simulink model "sampleModel1492_3_sub"  (R2023a)
settings: Solver=VariableStepAuto  StartTime=0.0  StopTime=10.0  RelTol=1e-3
libraries: hdlsllib x5, simulink x1
settings Model: Creator=user1  LastModifiedBy=user1
settings OptimizationCC: BlockReduction=off  ConditionallyExecuteInputs=off

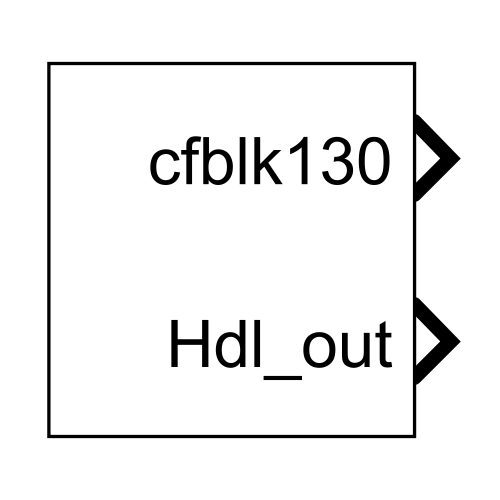
[thumbnail: Simulink's stored preview of the top-level diagram]
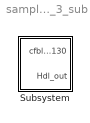
== system sampleModel1492_3_sub ==
  Subsystem : Subsystem

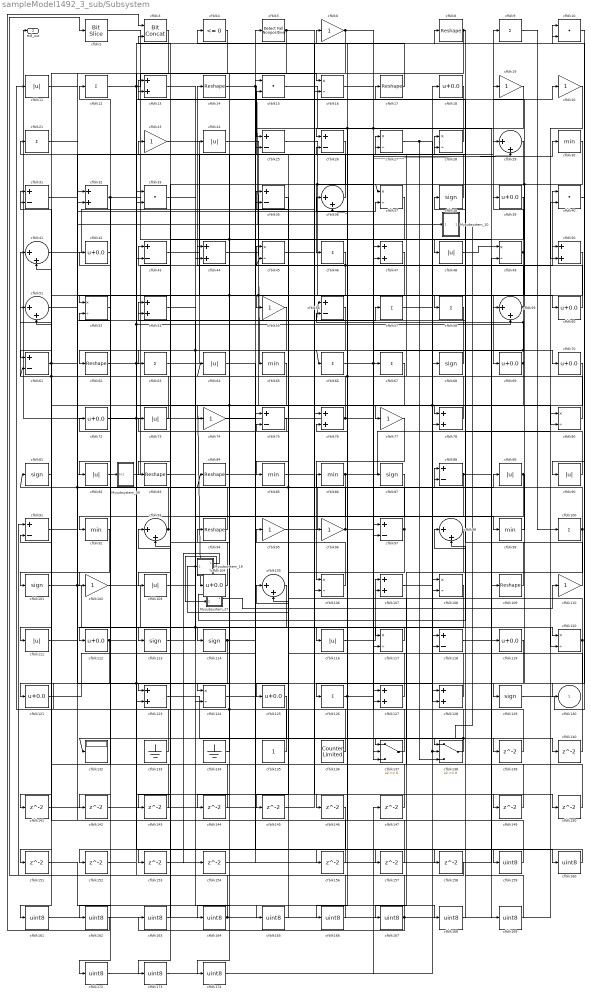
== system sampleModel1492_3_sub/Subsystem ==
  Mysubsystem_10 : Subsystem  TreatAsAtomicUnit=on  RTWFcnName=Mysubsystem_10
      settings: RTWFcnNameOpts=User specified  RTWFileNameOpts=Use function name
  Mysubsystem_19 : Subsystem  TreatAsAtomicUnit=on  RTWFcnName=Mysubsystem_19
      settings: RTWFcnNameOpts=User specified  RTWFileNameOpts=Use function name
  Mysubsystem_27 : Subsystem  TreatAsAtomicUnit=on  RTWFcnName=Mysubsystem_27
      settings: RTWFcnNameOpts=User specified  RTWFileNameOpts=Use function name
  Mysubsystem_39 : Subsystem  TreatAsAtomicUnit=on  RTWFcnName=Mysubsystem_39
      settings: RTWFcnNameOpts=User specified  RTWFileNameOpts=Use function name
  cfblk{10,15,33,40} (4 alike) : DotProduct  OutDataTypeStr=uint8
  cfblk{9,12,21,46,57..58,63,66..67,100,126} (11 alike) : Sum  Inputs=+  OutDataTypeStr=uint8
  cfblk{38,68,81,87,101,113..114,129} (8 alike) : Signum
  cfblk{6,19..20,23,55,74,77,95..96,102,110} (11 alike) : Gain  OutDataTypeStr=uint8
  cfblk{11,24,48,64,73,82,89..90,103,111,116} (11 alike) : Abs  OutDataTypeStr=uint8  SaturateOnIntegerOverflow=off
  cfblk{18,39,42,60,69..70,72,104,112,119,121,125} (12 alike) : Bias  Bias=0.0  SaturateOnIntegerOverflow=off
  cfblk{29,36,41,51,59,93,98,105} (8 alike) : Sum  Inputs=|++  OutDataTypeStr=uint8
  cfblk{16,27..28,37,45,49,52,80,106,108,117,120,124} (13 alike) : Product  Inputs=*/  OutDataTypeStr=uint8  RndMeth=Zero  SaturateOnIntegerOverflow=on
  cfblk{13,32,44,47,50,53,76,78,107,123,127..128} (12 alike) : Sum  OutDataTypeStr=uint8
  cfblk{8,14,17,62,83..84,94,109} (8 alike) : Reshape
  cfblk{25..26,31,35,43,56,61,75,88,91,97,118} (12 alike) : Sum  Inputs=+-  OutDataTypeStr=uint8
  cfblk132 : Display
  cfblk133 : Ground
  cfblk134 : Ground
  cfblk135 : Constant  OutDataTypeStr=uint8  SampleTime=-1
  cfblk136 : hdlsllib/Sources/Counter Limited  uplimit=7  tsamp=-1
  cfblk137 : Switch  OutDataTypeStr=uint8  SaturateOnIntegerOverflow=off  InputSameDT=off
  cfblk138 : Switch  OutDataTypeStr=uint8  SaturateOnIntegerOverflow=off  InputSameDT=off
  cfblk{139..147,149..154,156..158} (18 alike) : Delay  SampleTime=1
  cfblk{159..169,172..174} (14 alike) : DataTypeConversion  OutDataTypeStr=uint8  SaturateOnIntegerOverflow=off  RndMeth=Floor
  cfblk2 : hdlsllib/Logic and Bit Operations/Bit Slice  lidx=7  ridx=0
  cfblk3 : hdlsllib/Logic and Bit Operations/Bit Concat  numInputs=2
  cfblk{30,65,85..86,92,99} (6 alike) : MinMax  OutDataTypeStr=uint8
  cfblk4 : hdlsllib/Logic and Bit Operations/Compare To Zero  relop=<=  OutDataTypeStr=uint8
  cfblk5 : hdlsllib/Logic and Bit Operations/Detect Fall Nonpositive  vinit=0  OutDataTypeStr=uint8
  cfblk130 : Outport  OutDataTypeStr=uint8  VectorParamsAs1DForOutWhenUnconnected=off
  Hdl_out : Outport  Port=2  OutDataTypeStr=uint8
  wires:
  cfblk73/1 -> cfblk41/1
  cfblk9/1 -> cfblk100/1
  cfblk102/1 -> cfblk114/1
  cfblk44/1 -> cfblk97/2, cfblk77/1
  cfblk25/1 -> cfblk87/1, cfblk58/1
  cfblk75/1 -> cfblk43/1
  cfblk6/1 -> cfblk70/1, cfblk61/1
  cfblk61/1 -> cfblk28/1, cfblk121/1
  cfblk36/1 -> cfblk21/1
  cfblk76/1 -> Hdl_out/1, cfblk31/2, cfblk29/2, cfblk67/1
  cfblk50/1 -> cfblk52/1
  cfblk112/1 -> cfblk88/2, cfblk11/1
  cfblk93/1 -> cfblk23/1, cfblk12/1
  cfblk29/1 -> cfblk46/1
  cfblk30/1 -> cfblk59/1, cfblk37/1
  cfblk19/1 -> cfblk26/1
  cfblk46/1 -> cfblk45/2, cfblk144/1, cfblk111/1
  cfblk63/1 -> cfblk27/1
  cfblk133/1 -> cfblk51/1
  cfblk42/1 -> cfblk82/1
  cfblk120/1 -> cfblk45/1, cfblk126/1
  cfblk72/1 -> cfblk156/1, cfblk59/2, cfblk20/1
  cfblk32/1 -> cfblk44/2, cfblk112/1
  cfblk114/1 -> cfblk160/1, cfblk151/1, cfblk123/2
  cfblk18/1 -> cfblk137/3, cfblk166/1, cfblk35/2
  cfblk59/1 -> cfblk25/2, cfblk78/1, cfblk56/1
  cfblk95/1 -> cfblk89/1
  cfblk48/1 -> cfblk49/1
  cfblk77/1 -> cfblk106/1
  cfblk13/1 -> cfblk158/1, cfblk117/2
  cfblk15/1 -> cfblk119/1
  cfblk105/1 -> cfblk164/1
  cfblk94/1 -> cfblk31/1, cfblk61/2
  cfblk82/1 -> cfblk40/1
  cfblk27/1 -> cfblk138/3, cfblk68/1
  cfblk92/1 -> cfblk101/1
  cfblk4/1 -> cfblk32/2
  cfblk121/1 -> cfblk5/1
  cfblk89/1 -> cfblk137/2, cfblk129/1
  cfblk111/1 -> cfblk84/1, cfblk37/2
  cfblk87/1 -> cfblk96/1
  cfblk127/1 -> cfblk75/2
  cfblk2/1 -> cfblk109/1
  cfblk69/1 -> cfblk28/2, cfblk66/1, cfblk78/2, cfblk104/1
  cfblk123/1 -> cfblk138/1
  cfblk12/1 -> cfblk80/2, cfblk16/1
  cfblk116/1 -> cfblk107/1
  cfblk104/1 -> cfblk73/1
  cfblk90/1 -> cfblk38/1
  cfblk8/1 -> cfblk174/1, Mysubsystem_27/1(In1)
  cfblk101/1 -> cfblk120/2, cfblk116/1
  cfblk49/1 -> cfblk118/2, cfblk9/1
  cfblk88/1 -> cfblk103/1, cfblk50/1
  cfblk24/1 -> cfblk97/1
  cfblk81/1 -> cfblk51/2
  cfblk14/1 -> cfblk60/1, cfblk65/1
  cfblk74/1 -> cfblk15/1
  cfblk56/1 -> cfblk124/2, cfblk83/1
  cfblk43/1 -> cfblk69/1
  cfblk128/1 -> cfblk36/1
  cfblk135/1 -> cfblk94/1
  cfblk23/1 -> cfblk128/1
  cfblk113/1 -> cfblk88/1
  cfblk62/1 -> cfblk149/1, cfblk10/2, cfblk14/1
  cfblk66/1 -> cfblk30/1
  cfblk38/1 -> cfblk15/2
  cfblk3/1 -> cfblk161/1
  cfblk110/1 -> cfblk53/1
  cfblk119/1 -> cfblk137/1
  cfblk5/1 -> cfblk150/1, cfblk33/2
  cfblk52/1 -> cfblk92/1
  cfblk41/1 -> cfblk17/1
  cfblk91/1 -> cfblk57/1
  cfblk65/1 -> cfblk141/1, cfblk124/1
  cfblk31/1 -> cfblk55/1
  cfblk60/1 -> cfblk39/1
  cfblk26/1 -> cfblk93/2
  cfblk107/1 -> cfblk118/1
  cfblk129/1 -> cfblk10/1
  cfblk137/1 -> cfblk76/2
  cfblk126/1 -> cfblk6/1, cfblk47/2
  cfblk80/1 -> cfblk27/2
  cfblk100/1 -> cfblk117/1, cfblk35/1, cfblk81/1
  cfblk109/1 -> cfblk13/1
  cfblk103/1 -> cfblk56/2
  cfblk138/1 -> cfblk132/1, cfblk42/1
  cfblk57/1 -> cfblk120/1
  cfblk117/1 -> cfblk113/1
  cfblk10/1 -> cfblk90/1
  cfblk17/1 -> cfblk4/1
  cfblk39/1 -> cfblk123/1, cfblk74/1
  cfblk134/1 -> cfblk44/1
  cfblk68/1 -> cfblk62/1
  cfblk45/1 -> cfblk8/1
  cfblk51/1 -> cfblk127/2
  cfblk99/1 -> cfblk19/1
  cfblk98/1 -> cfblk167/1
  cfblk97/1 -> cfblk125/1, cfblk72/1
  cfblk53/1 -> cfblk99/1
  cfblk78/1 -> cfblk64/1, cfblk36/2
  cfblk106/1 -> cfblk95/1
  cfblk96/1 -> cfblk29/1, cfblk86/1
  cfblk136/1 -> cfblk24/1, cfblk13/2
  cfblk33/1 -> cfblk128/2
  cfblk40/1 -> cfblk130/1
  cfblk28/1 -> cfblk25/1
  cfblk16/1 -> cfblk48/1
  cfblk20/1 -> cfblk50/2
  cfblk47/1 -> cfblk63/1
  cfblk85/1 -> cfblk106/2
  cfblk58/1 -> cfblk85/1
  cfblk86/1 -> cfblk40/2, cfblk102/1
  cfblk139/1 -> cfblk127/1
  cfblk124/1 -> cfblk140/1
  cfblk140/1 -> cfblk47/1
  cfblk141/1 -> cfblk16/2
  cfblk67/1 -> cfblk142/1
  cfblk142/1 -> cfblk43/2
  cfblk55/1 -> cfblk143/1
  cfblk143/1 -> cfblk91/2
  cfblk144/1 -> cfblk52/2
  cfblk37/1 -> cfblk145/1
  cfblk145/1 -> cfblk76/1
  cfblk84/1 -> cfblk146/1
  cfblk147/1 -> cfblk53/2
  cfblk149/1 -> cfblk107/2
  cfblk150/1 -> cfblk93/1
  cfblk70/1 -> cfblk153/1
  cfblk153/1 -> cfblk49/2
  cfblk154/1 -> cfblk75/1
  cfblk156/1 -> cfblk32/1
  cfblk64/1 -> cfblk157/1
  cfblk157/1 -> cfblk41/2
  cfblk158/1 -> cfblk2/1
  cfblk152/1 -> cfblk159/1
  cfblk159/1 -> cfblk26/2
  cfblk160/1 -> cfblk152/1
  cfblk161/1 -> cfblk18/1, cfblk138/2
  cfblk146/1 -> cfblk162/1
  cfblk162/1 -> cfblk3/1
  cfblk163/1 -> cfblk3/2
  cfblk164/1 -> cfblk91/1, cfblk80/1
  cfblk83/1 -> cfblk165/1
  cfblk165/1 -> cfblk105/1
  cfblk166/1 -> cfblk105/2
  cfblk167/1 -> cfblk33/1, cfblk163/1
  cfblk151/1 -> cfblk168/1
  cfblk168/1 -> cfblk98/1
  cfblk118/1 -> cfblk169/1
  cfblk169/1 -> cfblk98/2
  cfblk108/1 -> cfblk172/1
  cfblk172/1 -> cfblk147/1
  cfblk125/1 -> cfblk173/1
  cfblk173/1 -> cfblk108/1
  cfblk174/1 -> cfblk108/2
  cfblk11/1 -> Mysubsystem_10/1(In1)
  Mysubsystem_10/1(Out1) -> cfblk139/1
  cfblk35/1 -> Mysubsystem_19/1(In1)
  Mysubsystem_19/1(Out1) -> cfblk154/1
  Mysubsystem_19/2(Out2) -> Mysubsystem_27/2(In2)
  Mysubsystem_27/1(Out1) -> cfblk110/1
  cfblk21/1 -> Mysubsystem_39/1(In1)

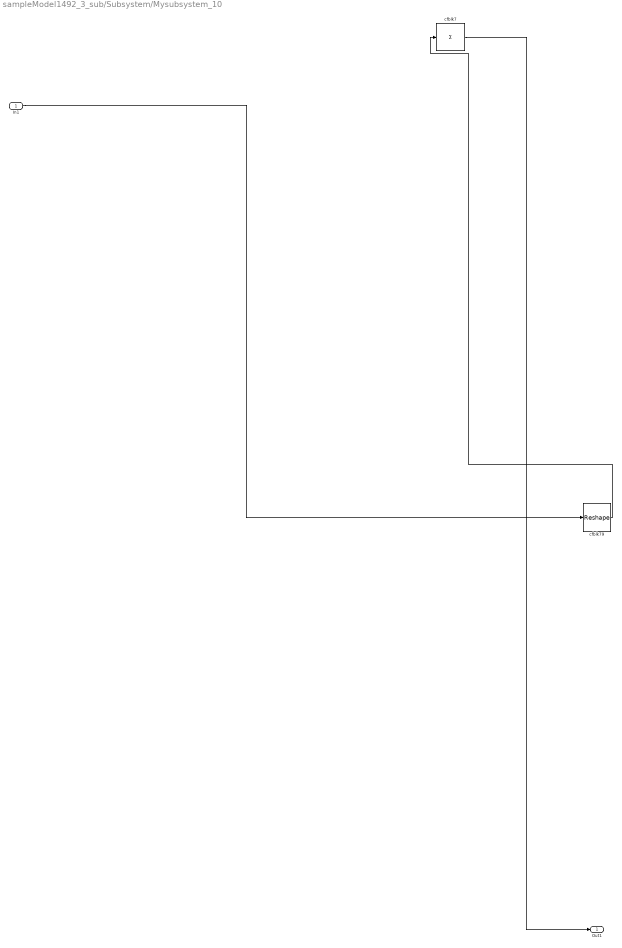
== system sampleModel1492_3_sub/Subsystem/Mysubsystem_10 ==
  In1 : Inport
  cfblk7 : Sum  Inputs=+
  cfblk79 : Reshape
  Out1 : Outport
  wires:
  cfblk7/1 -> Out1/1
  In1/1 -> cfblk79/1
  cfblk79/1 -> cfblk7/1

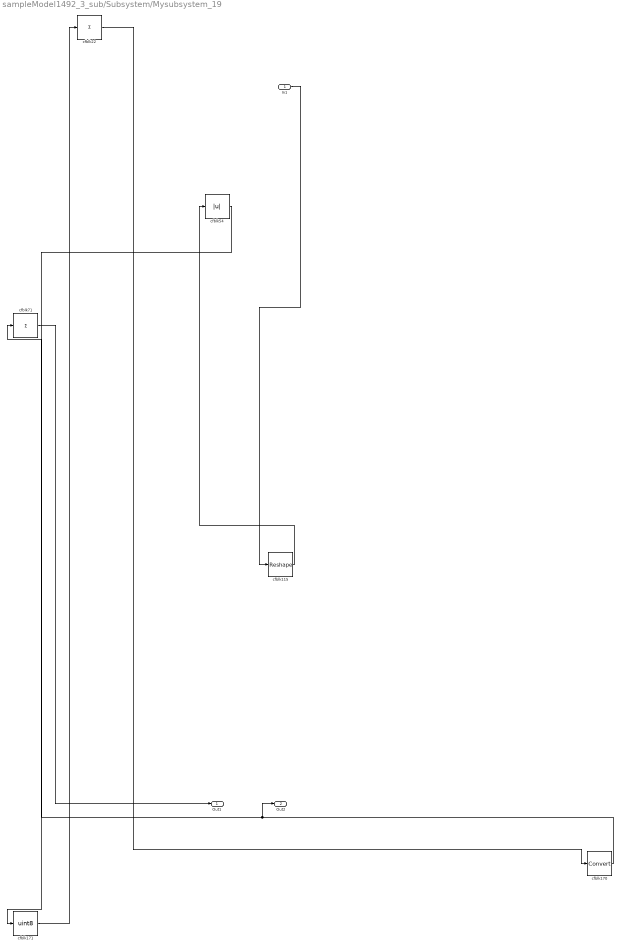
== system sampleModel1492_3_sub/Subsystem/Mysubsystem_19 ==
  In1 : Inport
  cfblk115 : Reshape
  cfblk170 : DataTypeConversion  SaturateOnIntegerOverflow=off  RndMeth=Floor
  cfblk171 : DataTypeConversion  OutDataTypeStr=uint8  SaturateOnIntegerOverflow=off  RndMeth=Floor
  cfblk22 : Sum  Inputs=+
  cfblk54 : Abs  SaturateOnIntegerOverflow=off
  cfblk71 : Sum  Inputs=+
  Out1 : Outport
  Out2 : Outport  Port=2
  wires:
  In1/1 -> cfblk115/1
  cfblk171/1 -> cfblk22/1
  cfblk54/1 -> cfblk171/1
  cfblk71/1 -> Out1/1
  cfblk170/1 -> cfblk71/1, Out2/1
  cfblk115/1 -> cfblk54/1
  cfblk22/1 -> cfblk170/1

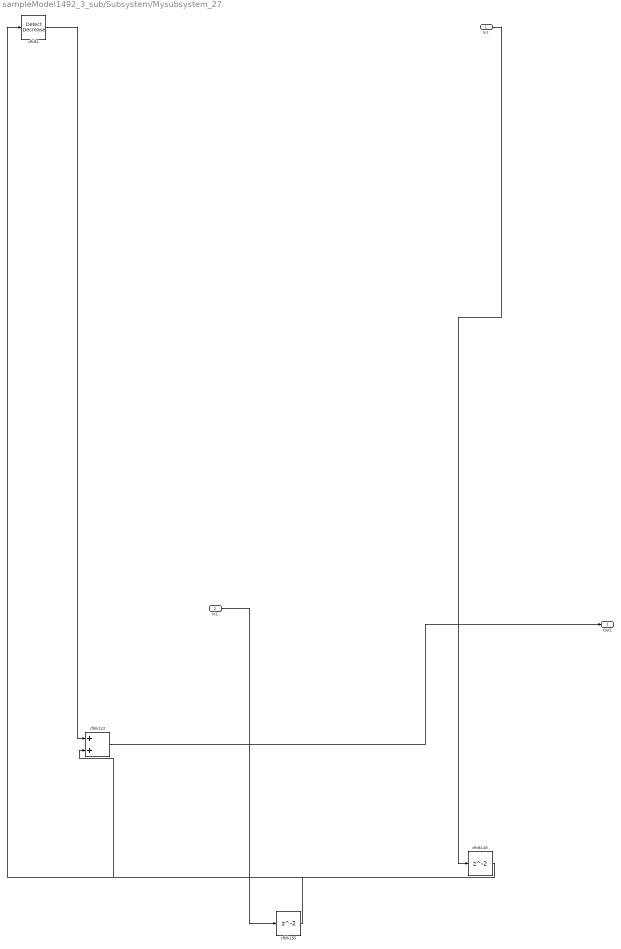
== system sampleModel1492_3_sub/Subsystem/Mysubsystem_27 ==
  In1 : Inport
  In2 : Inport  Port=2
  cfblk1 : simulink/Logic and Bit Operations/Detect Decrease  vinit=0.0  OutDataTypeStr=boolean
      settings: LibrarySourceBlock=|
      | hdlsllib/Logic and Bit
      | Operations/Detect
      | Decrease
  cfblk122 : Sum
  cfblk148 : Delay  SampleTime=1
  cfblk155 : Delay  SampleTime=1
  Out1 : Outport
  wires:
  cfblk1/1 -> cfblk122/1
  In1/1 -> cfblk148/1
  In2/1 -> cfblk155/1
  cfblk122/1 -> Out1/1
  cfblk155/1 -> cfblk122/2
  cfblk148/1 -> cfblk1/1

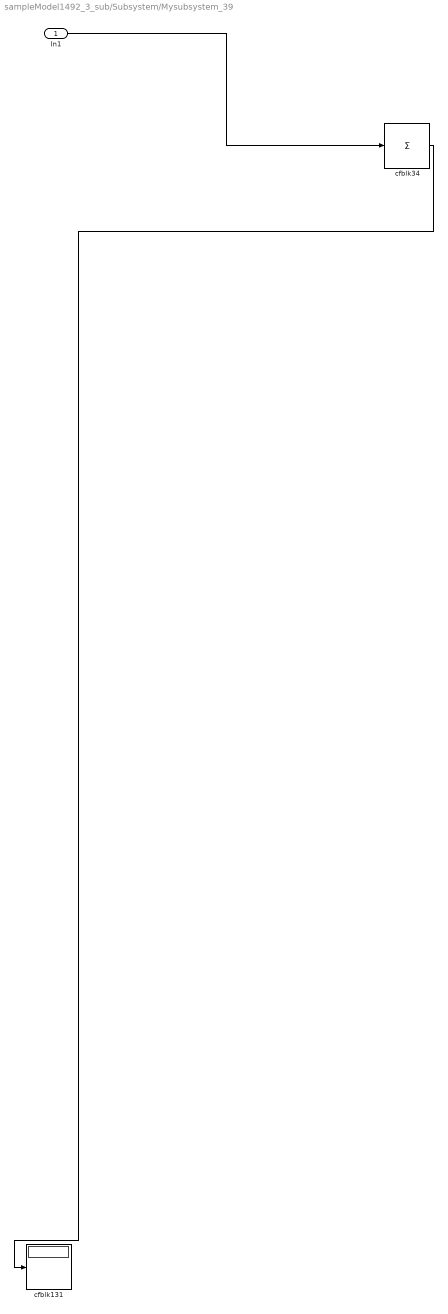
== system sampleModel1492_3_sub/Subsystem/Mysubsystem_39 ==
  In1 : Inport
  cfblk131 : Display
  cfblk34 : Sum  Inputs=+
  wires:
  In1/1 -> cfblk34/1
  cfblk34/1 -> cfblk131/1
